simulink model "PumpAdditionalIntegrationParallel_QuadChar"  (R2018b)
settings: Solver=ode45  StartTime=0.0  StopTime=400  MaxStep=5  RelTol=1e-3  EnableMultiTasking=on
undefined symbols (not defined in the file): DiameterLastPiece, DPConstant, DPLinear, DPQuadratic, ID, MassFlow, path_carnot, Pressure, Temperature, Water
libraries: carnot x12, simulink x4
settings Model: Creator=drhf  LastModifiedBy=drhf
settings DataIOCC: SaveFormat=Array  SignalLoggingSaveFormat=ModelDataLogs
settings OptimizationCC: ExpressionDepthLimit=2147483647  LifeSpan=inf
settings DebuggingCC: UnderspecifiedInitializationDetection=Classic  MergeDetectMultiDrivingBlocksExec=none  SolverPrmCheckMsg=warning  StateNameClashWarn=warning  SFUnexpectedBacktrackingDiag=warning  SFNoUnconditionalDefaultTransitionDiag=warning  SFExecutionAtInitializationDiag=none
settings HardwareCC: ProdBitPerPointer=32  ProdBitPerSizeT=32  ProdBitPerPtrDiffT=32  ProdLargestAtomicFloat=None  ProdIntDivRoundTo=Undefined  ProdEndianess=Unspecified  ProdWordSize=32  ProdHWDeviceType=32-bit Generic
settings ModelReferenceCC: PropagateSignalLabelsOutOfModel=off
settings SFSimCC: SimUseLocalCustomCode=off
settings RTWCC: RTWUseLocalCustomCode=off
settings CodeAppCC: StateflowObjectComments=on
settings GRTTargetCC: TargetLangStandard=C89/C90 (ANSI)  GeneratePreprocessorConditionals=Disable all  CombineOutputUpdateFcns=off  GRTInterface=on
settings ConfigComp: CovMetricSettings=dw  CovHtmlReporting=on  CovSaveCumulativeToWorkspaceVar=on  CovSaveSingleToWorkspaceVar=on  CovExternalEMLEnable=off

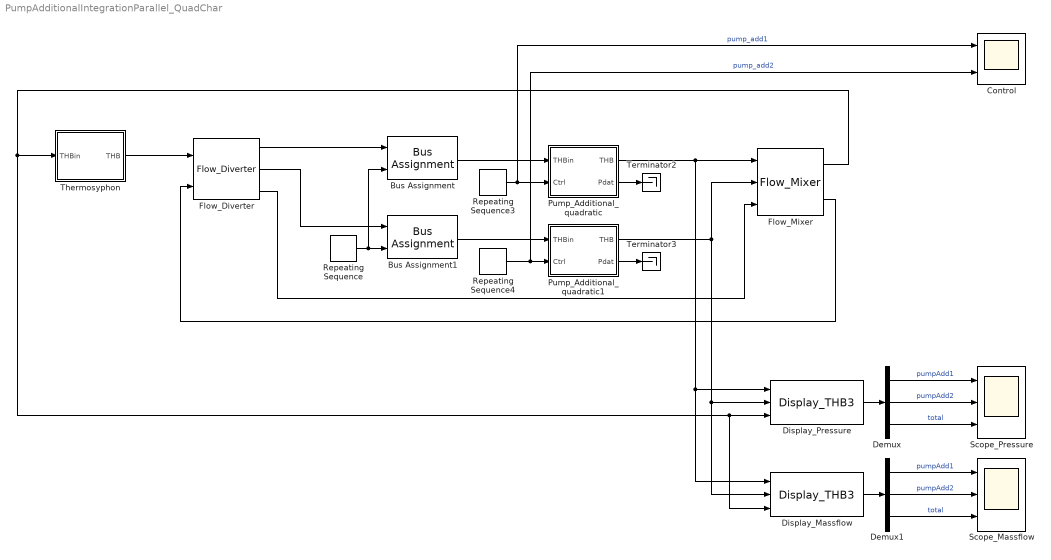
== system PumpAdditionalIntegrationParallel_QuadChar ==
  Bus Assignment : BusAssignment  AssignedSignals=DPQuadratic
  Bus Assignment1 : BusAssignment  AssignedSignals=DPQuadratic
  Control : Scope  NumInputPorts=2
  Demux : Demux  Outputs=3
  Demux1 : Demux  Outputs=3
  Display_Massflow : carnot/Outputs/Display_THB3  t=off  m=on  p=off  id=off  mix=off  d=off
  Display_Pressure : carnot/Outputs/Display_THB3  t=off  m=off  p=on  id=off  mix=off  d=off
  Flow_Diverter : carnot/Hydraulics/Flow_Diverter
  Flow_Mixer : carnot/Hydraulics/Flow_Mixer
  Pump_Additional_quadratic : Subsystem  AncestorBlock=carnot/Hydraulics/Pump_Additional  mask(Pump Additional){Tini=20, PathName=fullfile(path_carnot('libsl'), 'Hydraulics', 'Pump_Main', 'parameter_set'), FileName='Pump6m.mat', userPath=off, userParam=off, a0=60000, a1=-43200, a2=0, dia=0.025, UA=1, mcp=4182, e0=50, e1=28.8, e2=-10.368}
      mask prompts: Tini "Ambient temperature for losses and initial temperture in °C"; PathName "Path"; FileName "Parameter set"; userPath "Edit path and name of parameter set"; userParam "User defined parameters"; a0 "a0: pump head in [Pa] (pressure increase at zero flow)"; a1 "a1: pump characteristic linear coefficient [Pa*s/kg]"; a2 "a2: pump characteristic quadratic coefficient [Pa*(s/kg)²]"; dia "Diameter at in- and outlet [m]"; UA "UA: thermal loss coefficient in W/K"; mcp "mcp: thermal capacity of the node in J/K"; e0 "e0: constant coefficient in W"; e1 "e1: linear coefficient in W*s/kg"; e2 "e2: quadratic coefficient in W*(s/kg)²"
      mask help:
      | This is an additional pump in a circuit. Every circuit must have exactly ONE 'Pump_Main'. It may have several 'Pump_Additional' blocks. The pump adds pump_head to the pressure drop of the circuit dp_circuit:
      |     dp_circuit = c + l*mdot + q*(mdot)²
      |     pump_head_ = a0*Ctrl² + a1*Ctrl*mdot +a2*mdot²
      |     dp_total = pump_head - dp_circuit
      |     p1 = system_pressure + (a0*Ctrl² - c) + (a1*Ctrl - l) * mdot + (a2-q)*(mdot)²
      | with
      |   Ctrl : Control signal input [0..1]
      | Note: Pump_Additional uses the parameters sets as Pump_Main.
      mask init:
      | % callback to set parameters of model
      | [ok, param] = CarnotCallbacks_PumpAdditional('SetParameters',gcbh,PathName,FileName);
      mask Help: web(fullfile(path_carnot('help'),'Pump_Main.html'),'-helpbrowser')
      mask TypeOptions Tini: ThermalNodeTHB/Tini
      mask Callback userPath: [ok, param] = CarnotCallbacks_PumpAdditional('UserEdit',gcbh);
      mask Callback userParam: [ok, param] = CarnotCallbacks_PumpAdditional('UserEdit',gcbh);
      mask TypeOptions a0: PumpHead/Gain
      mask TypeOptions a1: PumpLinear/Gain
      mask TypeOptions a2: PumpQuadratic/Value
      mask TypeOptions dia: dia/Value
      mask TypeOptions UA: ThermalNodeTHB/UA
      mask TypeOptions mcp: ThermalNodeTHB/mcp
      mask TypeOptions e0: ElectricConsumptionPump/e0
      mask TypeOptions e1: ElectricConsumptionPump/e1
      mask TypeOptions e2: ElectricConsumptionPump/e2
      mask DialogControl ParameterGroupFile Prompt: Picking a parameter set
      mask DialogControl Control1 Prompt: Carnot public data
      mask DialogControl Control1 Callback: [ok, file] = CarnotCallbacks_PumpAdditional('GetFilename',gcbh,'public');
      mask DialogControl Control3 Prompt: Carnot internal data
      mask DialogControl Control3 Callback: [ok, file] = CarnotCallbacks_PumpAdditional('GetFilename',gcbh,'internal');
      mask DialogControl Control4 Prompt: Selected path
      mask DialogControl Control4 Callback: [ok, file] = CarnotCallbacks_PumpAdditional('GetFilename',gcbh,'selected');
      mask DialogControl PrameterGroupUser Prompt: Parameter Values
      mask DialogControl Container9 Prompt: Hydraulic
      mask DialogControl Container7 Prompt: Thermal
      mask DialogControl Control9 Prompt: Thermal node for temperature:  mcp * dTnode/dt = UA*(Tamb-Tnode) + mdot*cp_in*(Tin-Tnode)
      mask DialogControl Container12 Prompt: Electric
      mask DialogControl Control7 Prompt: Power consumption  Pel = e0 + e1*mdot + e2*mdot²
      mask DialogControl Control5 Prompt: Save in Carnot internal data
      mask DialogControl Control5 Callback: [ok, param] = CarnotCallbacks_PumpAdditional('SaveFilename',gcbh,'internal','B');
      mask DialogControl Control6 Prompt: Save in selected path
      mask DialogControl Control6 Callback: [ok, param] = CarnotCallbacks_PumpAdditional('SaveFilename',gcbh,'selected','B');
      mask Display:
      | % user defined picture file
      | picfile = fullfile(path_carnot('intlibsl'), ...
      |         'Hydraulics', 'Pump_Additional', 'PumpAdditional.jpg');
      | 
      | pic = false;
      | if ~BlockIsInCarnotLibrary    % if not located in library any more
      |     if exist(picfile,'file') % show internal picture if defined
      |         image(imread(picfile), [0.2, 0, 0.6, 1])
      |         set_param(gcb, 'BackgroundColor', 'White')
      |         pic = true;
      |     end
      | end
      | if ~pic    % show public picture
      |     set_param(gcb, 'BackgroundColor', 'green')
      |     plot(0,0,1,1,[40,70,40,30,30,40,60,70,70,60,40]/100, ...
      |         [70,50,30,40,60,70,70,60,40,30,30]/100)
      |     disp('add')
      | end
  Pump_Additional_quadratic1 : Subsystem  AncestorBlock=carnot/Hydraulics/Pump_Additional  mask(Pump Additional){Tini=20, PathName=fullfile(path_carnot('libsl'), 'Hydraulics', 'Pump_Main', 'parameter_set'), FileName='Pump6m.mat', userPath=off, userParam=off, a0=60000, a1=-43200, a2=0, dia=0.025, UA=1, mcp=4182, e0=50, e1=28.8, e2=-10.368}
      mask prompts: Tini "Ambient temperature for losses and initial temperture in °C"; PathName "Path"; FileName "Parameter set"; userPath "Edit path and name of parameter set"; userParam "User defined parameters"; a0 "a0: pump head in [Pa] (pressure increase at zero flow)"; a1 "a1: pump characteristic linear coefficient [Pa*s/kg]"; a2 "a2: pump characteristic quadratic coefficient [Pa*(s/kg)²]"; dia "Diameter at in- and outlet [m]"; UA "UA: thermal loss coefficient in W/K"; mcp "mcp: thermal capacity of the node in J/K"; e0 "e0: constant coefficient in W"; e1 "e1: linear coefficient in W*s/kg"; e2 "e2: quadratic coefficient in W*(s/kg)²"
      mask help:
      | This is an additional pump in a circuit. Every circuit must have exactly ONE 'Pump_Main'. It may have several 'Pump_Additional' blocks. The pump adds pump_head to the pressure drop of the circuit dp_circuit:
      |     dp_circuit = c + l*mdot + q*(mdot)²
      |     pump_head_ = a0*Ctrl² + a1*Ctrl*mdot +a2*mdot²
      |     dp_total = pump_head - dp_circuit
      |     p1 = system_pressure + (a0*Ctrl² - c) + (a1*Ctrl - l) * mdot + (a2-q)*(mdot)²
      | with
      |   Ctrl : Control signal input [0..1]
      | Note: Pump_Additional uses the parameters sets as Pump_Main.
      mask init:
      | % callback to set parameters of model
      | [ok, param] = CarnotCallbacks_PumpAdditional('SetParameters',gcbh,PathName,FileName);
      mask Help: web(fullfile(path_carnot('help'),'Pump_Main.html'),'-helpbrowser')
      mask TypeOptions Tini: ThermalNodeTHB/Tini
      mask Callback userPath: [ok, param] = CarnotCallbacks_PumpAdditional('UserEdit',gcbh);
      mask Callback userParam: [ok, param] = CarnotCallbacks_PumpAdditional('UserEdit',gcbh);
      mask TypeOptions a0: PumpHead/Gain
      mask TypeOptions a1: PumpLinear/Gain
      mask TypeOptions a2: PumpQuadratic/Value
      mask TypeOptions dia: dia/Value
      mask TypeOptions UA: ThermalNodeTHB/UA
      mask TypeOptions mcp: ThermalNodeTHB/mcp
      mask TypeOptions e0: ElectricConsumptionPump/e0
      mask TypeOptions e1: ElectricConsumptionPump/e1
      mask TypeOptions e2: ElectricConsumptionPump/e2
      mask DialogControl ParameterGroupFile Prompt: Picking a parameter set
      mask DialogControl Control1 Prompt: Carnot public data
      mask DialogControl Control1 Callback: [ok, file] = CarnotCallbacks_PumpAdditional('GetFilename',gcbh,'public');
      mask DialogControl Control3 Prompt: Carnot internal data
      mask DialogControl Control3 Callback: [ok, file] = CarnotCallbacks_PumpAdditional('GetFilename',gcbh,'internal');
      mask DialogControl Control4 Prompt: Selected path
      mask DialogControl Control4 Callback: [ok, file] = CarnotCallbacks_PumpAdditional('GetFilename',gcbh,'selected');
      mask DialogControl PrameterGroupUser Prompt: Parameter Values
      mask DialogControl Container9 Prompt: Hydraulic
      mask DialogControl Container7 Prompt: Thermal
      mask DialogControl Control9 Prompt: Thermal node for temperature:  mcp * dTnode/dt = UA*(Tamb-Tnode) + mdot*cp_in*(Tin-Tnode)
      mask DialogControl Container12 Prompt: Electric
      mask DialogControl Control7 Prompt: Power consumption  Pel = e0 + e1*mdot + e2*mdot²
      mask DialogControl Control5 Prompt: Save in Carnot internal data
      mask DialogControl Control5 Callback: [ok, param] = CarnotCallbacks_PumpAdditional('SaveFilename',gcbh,'internal','B');
      mask DialogControl Control6 Prompt: Save in selected path
      mask DialogControl Control6 Callback: [ok, param] = CarnotCallbacks_PumpAdditional('SaveFilename',gcbh,'selected','B');
      mask Display:
      | % user defined picture file
      | picfile = fullfile(path_carnot('intlibsl'), ...
      |         'Hydraulics', 'Pump_Additional', 'PumpAdditional.jpg');
      | 
      | pic = false;
      | if ~BlockIsInCarnotLibrary    % if not located in library any more
      |     if exist(picfile,'file') % show internal picture if defined
      |         image(imread(picfile), [0.2, 0, 0.6, 1])
      |         set_param(gcb, 'BackgroundColor', 'White')
      |         pic = true;
      |     end
      | end
      | if ~pic    % show public picture
      |     set_param(gcb, 'BackgroundColor', 'green')
      |     plot(0,0,1,1,[40,70,40,30,30,40,60,70,70,60,40]/100, ...
      |         [70,50,30,40,60,70,70,60,40,30,30]/100)
      |     disp('add')
      | end
  Repeating Sequence : simulink/Sources/Repeating Sequence  rep_seq_t=[0 200 200.1 400]  rep_seq_y="[1e3 1e3 1e3 1e3]      % [0 0 1 1]*(6e4/0.01)^2"
  Repeating Sequence3 : simulink/Sources/Repeating Sequence  rep_seq_t=[0 40 40.2 50 60 200]  rep_seq_y=[1 1 0 0 1 1]
  Repeating Sequence4 : simulink/Sources/Repeating Sequence  rep_seq_t=[0 90 95 200 200.1]  rep_seq_y=[0 0 1 1 0]
  Scope_Massflow : Scope  NumInputPorts=3
  Scope_Pressure : Scope  NumInputPorts=3
  Terminator2 : Terminator
  Terminator3 : Terminator
  Thermosyphon : Subsystem  AncestorBlock=carnot/Hydraulics/Thermosyphon  mask(thermosyphon){p0=3e5, dia=0.025, fluid_id=Water, mix=0, mix2=0, mix3=0, t1=1}
      mask prompts: p0 "static system pressure [Pa]"; dia "Diameter at in- and outlet [m]"; fluid_id "fluid"; mix "fluid mixture [0..1]"; mix2 "fluid mixture 2 [0..1]"; mix3 "fluid mixture 3 [0..1]"; t1 "Time constant of PT1 transfer function for massflow in s"
      mask help:
      | This block is a model of a "thermosyphon pump". Place it in natural convection systems as you would place a pump.
      | Assure that the sum of heights is zero. Otherwise the simulation will not start.
      | You may check the sum of heights by verifying the "Geodetic Height" in the THB at the inport of this block.
      | If the sum is not zero, the difference is displayed in the subsystem "Stop Simulation".
      | This model uses a Memory block to break an algebraic loop. Avoid using the variable-step solver ode15s or ode113 (see block help for details).
      | A unit delay block with a sample time ("time constant of the pump") limits the maximum stepsize.
      mask Help: web(fullfile(path_carnot('help'),'Thermosyphon.html'),'-helpbrowser')
      mask TypeOptions p0: basic_THB/p
      mask TypeOptions dia: basic_THB/dia
      mask TypeOptions fluid_id: basic_THB/fluid
      mask TypeOptions mix: basic_THB/mix
      mask TypeOptions mix2: basic_THB/mix2
      mask TypeOptions mix3: basic_THB/mix3
      mask TypeOptions t1: Transfer Fcn/t1
      mask DialogControl Container4 Prompt: Hydraulic
      mask Display: plot(0,0,100,100,[90,10],[80,90],[90,10],[70,80],[90,10],[20,10],[90,10],[30,20],[40,60,40,40],[60,50,40,60])
  wires:
  Pump_Additional_quadratic/2(Pdat) -> Terminator2/1
  Bus Assignment/1 -> Pump_Additional_quadratic/1(THBin)
  Display_Pressure/1 -> Demux/1
  Demux/1 -> Scope_Pressure/1  "pumpAdd1"
  Demux/2 -> Scope_Pressure/2  "pumpAdd2"
  Demux/3 -> Scope_Pressure/3  "total"
  Repeating Sequence3/1 -> Pump_Additional_quadratic/2(Ctrl), Control/1  "pump_add1"
  Repeating Sequence/1 -> Bus Assignment/2, Bus Assignment1/2
  Pump_Additional_quadratic1/2(Pdat) -> Terminator3/1
  Bus Assignment1/1 -> Pump_Additional_quadratic1/1(THBin)
  Repeating Sequence4/1 -> Pump_Additional_quadratic1/2(Ctrl), Control/2  "pump_add2"
  Pump_Additional_quadratic1/1(THB) -> Display_Massflow/2, Display_Pressure/2, Flow_Mixer/2
  Flow_Diverter/1 -> Bus Assignment/1
  Flow_Diverter/2 -> Bus Assignment1/1
  Flow_Diverter/3 -> Flow_Mixer/3
  Pump_Additional_quadratic/1(THB) -> Display_Massflow/1, Display_Pressure/1, Flow_Mixer/1
  Flow_Mixer/2 -> Flow_Diverter/2
  Display_Massflow/1 -> Demux1/1
  Demux1/1 -> Scope_Massflow/1  "pumpAdd1"
  Demux1/2 -> Scope_Massflow/2  "pumpAdd2"
  Demux1/3 -> Scope_Massflow/3  "total"
  Flow_Mixer/1 -> Display_Massflow/3, Display_Pressure/3, Thermosyphon/1(THBin)
  Thermosyphon/1(THB) -> Flow_Diverter/1

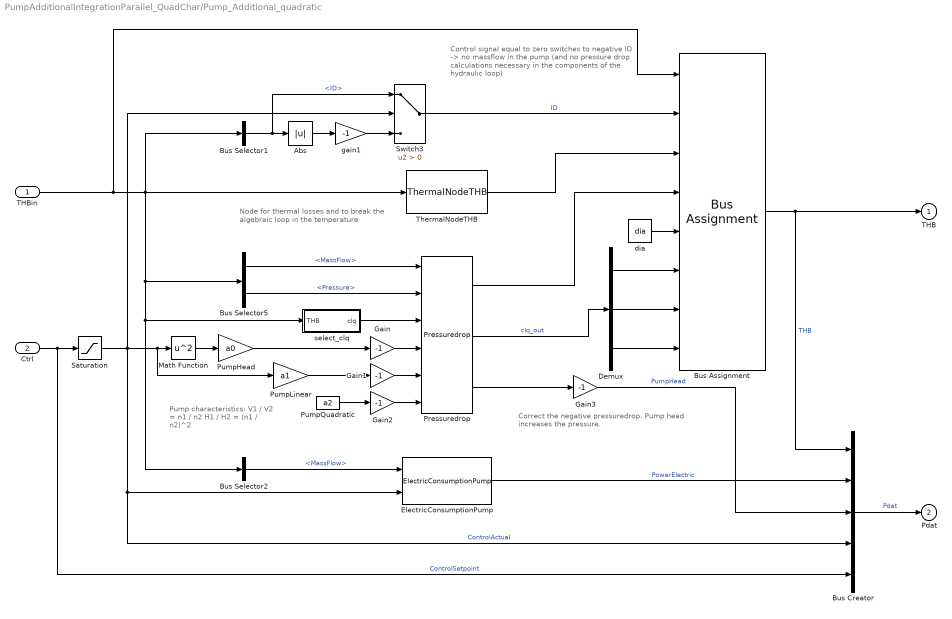
== system PumpAdditionalIntegrationParallel_QuadChar/Pump_Additional_quadratic ==
  note: Pump characteristics:
      | V1 / V2 = n1 / n2
      | H1 / H2 = (n1 / n2)^2
  note: Correct the negative pressuredrop.
      | Pump head increases the pressure.
  note: Control signal equal to zero switches
      | to negative ID -> no massflow in the
      | pump (and no pressure drop calculations
      | necessary in the components of the
      | hydraulic loop)
  note: Node for thermal losses and to break
      | the algebraic loop in the temperature
  THBin : Inport
  Ctrl : Inport  Port=2
  Abs : Abs
  Bus Assignment : BusAssignment  AssignedSignals=ID,Temperature,Pressure,DiameterLastPiece,DPConstant,DPLinear,DPQuadratic
  Bus Creator : BusCreator  Inputs=5
  Bus Selector1 : BusSelector  OutputSignals=ID
  Bus Selector2 : BusSelector  OutputSignals=MassFlow
  Bus Selector5 : BusSelector  OutputSignals=MassFlow,Pressure
  Demux : Demux  Outputs=3
  ElectricConsumptionPump : carnot/Basic/Hydraulics/ElectricConsumptionPump  e0=e0  e1=e1  e2=e2
  Gain{,1..3} (4 alike) : Gain  Gain=-1
  Math Function : Math  Operator=square  SaturateOnIntegerOverflow=on
  Pressuredrop : carnot/Basic/Pressure_Drop/Pressuredrop
  PumpHead : Gain  Gain=a0
  PumpLinear : Gain  Gain=a1
  PumpQuadratic : Constant  Value=a2
  Saturation : Saturate  UpperLimit=1  LowerLimit=0
  Switch3 : Switch  Criteria=u2 > Threshold  SaturateOnIntegerOverflow=on  InputSameDT=on
  ThermalNodeTHB : carnot/Basic/Thermal_Models/ThermalNodeTHB  UA=UA  mcp=mcp  Tini=Tini
  dia : Constant  Value=dia
  gain1 : Gain  Gain=-1  SaturateOnIntegerOverflow=on  OutDataTypeStr=Inherit: Same as input  ParamDataTypeStr=Inherit: Same as input
  select_clq : Subsystem
  THB : Outport
  Pdat : Outport  Port=2
  wires:
  Math Function/1 -> PumpHead/1
  Saturation/1 -> Switch3/2, Bus Creator/4, ElectricConsumptionPump/2, PumpLinear/1, Math Function/1  "ControlActual"
  Gain3/1 -> Bus Creator/3  "PumpHead"
  Pressuredrop/1 -> Bus Assignment/4
  Pressuredrop/2 -> Demux/1  "clq_out"
  Pressuredrop/3 -> Gain3/1
  Bus Assignment/1 -> THB/1, Bus Creator/1  "THB"
  Bus Selector2/1 -> ElectricConsumptionPump/1  "<MassFlow>"
  Bus Creator/1 -> Pdat/1  "Pdat"
  ElectricConsumptionPump/1 -> Bus Creator/2  "PowerElectric"
  Ctrl/1 -> Saturation/1, Bus Creator/5  "ControlSetpoint"
  Bus Selector1/1 -> Switch3/1, Abs/1  "<ID>"
  Abs/1 -> gain1/1
  gain1/1 -> Switch3/3
  Switch3/1 -> Bus Assignment/2  "ID"
  Bus Selector5/1 -> Pressuredrop/1  "<MassFlow>"
  dia/1 -> Bus Assignment/5
  THBin/1 -> Bus Selector1/1, Bus Selector2/1, select_clq/1(THB), Bus Selector5/1, ThermalNodeTHB/1, Bus Assignment/1
  PumpHead/1 -> Gain/1
  PumpLinear/1 -> Gain1/1
  PumpQuadratic/1 -> Gain2/1
  Demux/1 -> Bus Assignment/6
  Demux/2 -> Bus Assignment/7
  Demux/3 -> Bus Assignment/8
  ThermalNodeTHB/1 -> Bus Assignment/3
  select_clq/1(clq) -> Pressuredrop/3
  Bus Selector5/2 -> Pressuredrop/2  "<Pressure>"
  Gain/1 -> Pressuredrop/4
  Gain1/1 -> Pressuredrop/5
  Gain2/1 -> Pressuredrop/6

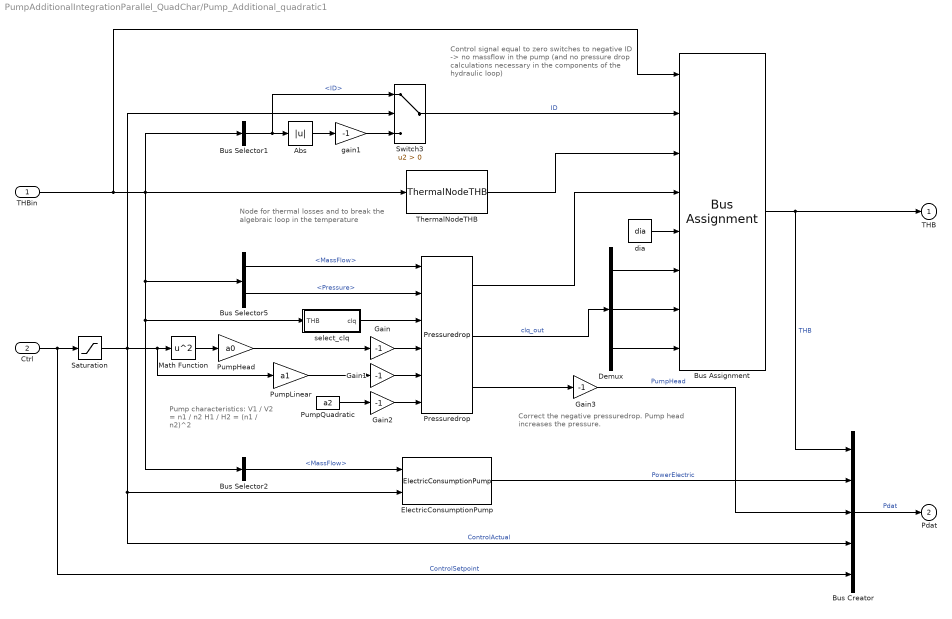
== system PumpAdditionalIntegrationParallel_QuadChar/Pump_Additional_quadratic1 ==
  note: Node for thermal losses and to break
      | the algebraic loop in the temperature
  note: Control signal equal to zero switches
      | to negative ID -> no massflow in the
      | pump (and no pressure drop calculations
      | necessary in the components of the
      | hydraulic loop)
  note: Correct the negative pressuredrop.
      | Pump head increases the pressure.
  note: Pump characteristics:
      | V1 / V2 = n1 / n2
      | H1 / H2 = (n1 / n2)^2
  THBin : Inport
  Ctrl : Inport  Port=2
  Abs : Abs
  Bus Assignment : BusAssignment  AssignedSignals=ID,Temperature,Pressure,DiameterLastPiece,DPConstant,DPLinear,DPQuadratic
  Bus Creator : BusCreator  Inputs=5
  Bus Selector1 : BusSelector  OutputSignals=ID
  Bus Selector2 : BusSelector  OutputSignals=MassFlow
  Bus Selector5 : BusSelector  OutputSignals=MassFlow,Pressure
  Demux : Demux  Outputs=3
  ElectricConsumptionPump : carnot/Basic/Hydraulics/ElectricConsumptionPump  e0=e0  e1=e1  e2=e2
  Gain{,1..3} (4 alike) : Gain  Gain=-1
  Math Function : Math  Operator=square  SaturateOnIntegerOverflow=on
  Pressuredrop : carnot/Basic/Pressure_Drop/Pressuredrop
  PumpHead : Gain  Gain=a0
  PumpLinear : Gain  Gain=a1
  PumpQuadratic : Constant  Value=a2
  Saturation : Saturate  UpperLimit=1  LowerLimit=0
  Switch3 : Switch  Criteria=u2 > Threshold  SaturateOnIntegerOverflow=on  InputSameDT=on
  ThermalNodeTHB : carnot/Basic/Thermal_Models/ThermalNodeTHB  UA=UA  mcp=mcp  Tini=Tini
  dia : Constant  Value=dia
  gain1 : Gain  Gain=-1  SaturateOnIntegerOverflow=on  OutDataTypeStr=Inherit: Same as input  ParamDataTypeStr=Inherit: Same as input
  select_clq : Subsystem
  THB : Outport
  Pdat : Outport  Port=2
  wires:
  Gain2/1 -> Pressuredrop/6
  Gain1/1 -> Pressuredrop/5
  Gain/1 -> Pressuredrop/4
  Bus Selector5/2 -> Pressuredrop/2  "<Pressure>"
  select_clq/1(clq) -> Pressuredrop/3
  ThermalNodeTHB/1 -> Bus Assignment/3
  Demux/3 -> Bus Assignment/8
  Demux/2 -> Bus Assignment/7
  Demux/1 -> Bus Assignment/6
  PumpQuadratic/1 -> Gain2/1
  PumpLinear/1 -> Gain1/1
  PumpHead/1 -> Gain/1
  THBin/1 -> Bus Assignment/1, ThermalNodeTHB/1, Bus Selector5/1, select_clq/1(THB), Bus Selector2/1, Bus Selector1/1
  dia/1 -> Bus Assignment/5
  Bus Selector5/1 -> Pressuredrop/1  "<MassFlow>"
  Switch3/1 -> Bus Assignment/2  "ID"
  gain1/1 -> Switch3/3
  Abs/1 -> gain1/1
  Bus Selector1/1 -> Abs/1, Switch3/1  "<ID>"
  Ctrl/1 -> Bus Creator/5, Saturation/1  "ControlSetpoint"
  ElectricConsumptionPump/1 -> Bus Creator/2  "PowerElectric"
  Bus Creator/1 -> Pdat/1  "Pdat"
  Bus Selector2/1 -> ElectricConsumptionPump/1  "<MassFlow>"
  Bus Assignment/1 -> Bus Creator/1, THB/1  "THB"
  Pressuredrop/3 -> Gain3/1
  Pressuredrop/2 -> Demux/1  "clq_out"
  Pressuredrop/1 -> Bus Assignment/4
  Gain3/1 -> Bus Creator/3  "PumpHead"
  Saturation/1 -> Math Function/1, PumpLinear/1, ElectricConsumptionPump/2, Bus Creator/4, Switch3/2  "ControlActual"
  Math Function/1 -> PumpHead/1

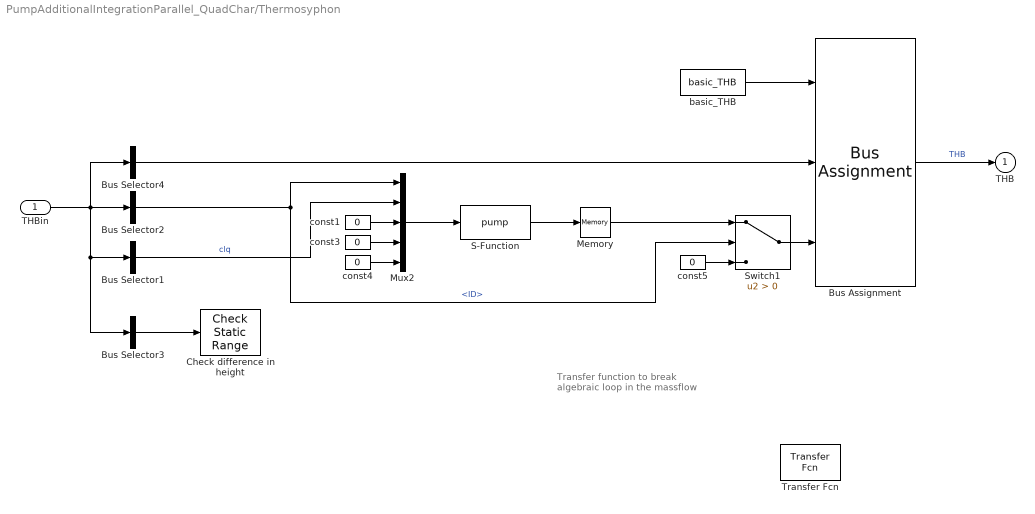
== system PumpAdditionalIntegrationParallel_QuadChar/Thermosyphon ==
  note: Transfer function to
      | break algebraic loop
      | in the massflow
  THBin : Inport
  Bus Assignment : BusAssignment  AssignedSignals=Temperature,MassFlow
  Bus Selector1 : BusSelector  OutputSignals=DPConstant,DPLinear,DPQuadratic  OutputAsBus=on
  Bus Selector2 : BusSelector  OutputSignals=ID
  Bus Selector3 : BusSelector  OutputSignals=GeodeticHeight  OutputAsBus=on
  Bus Selector4 : BusSelector  OutputSignals=Temperature  OutputAsBus=on
  Check difference in height : simulink/Model Verification/Check  Static Range  Description=-0.001 <= u <= 0.001  max=0.001  max_included=on  min=-0.001  min_included=on  enabled=on  stopWhenAssertionFail=on  export=off  icon=graphic
      settings: SourceProductName=Simulink  SourceProductBaseCode=SL
  Memory : Memory
  Mux2 : Mux  Inputs=5
  S-Function : S-Function  FunctionName=pump  SFunctionDeploymentMode=off  EnableBusSupport=off
  Switch1 : Switch  Criteria=u2 > Threshold  SaturateOnIntegerOverflow=on  InputSameDT=on
  Transfer Fcn : carnot/Hydraulics/Pump_Main/Transfer Fcn  t1=t1
  basic_THB : carnot/Basic/Hydraulics/basic_THB  t=20  mdot=0  p=p0  ID=Full Pressure Drop with Static Height  fluid=Water  mix=mix  mix2=mix2  mix3=mix3  dia=dia  hgt=0
  const{1,3..5} (4 alike) : Constant  Value=0
  THB : Outport
  wires:
  Bus Selector4/1 -> Bus Assignment/2
  Bus Selector2/1 -> Mux2/1, Switch1/2  "<ID>"
  Mux2/1 -> S-Function/1
  S-Function/1 -> Memory/1
  const3/1 -> Mux2/4
  const4/1 -> Mux2/5
  const1/1 -> Mux2/3
  Memory/1 -> Switch1/1
  const5/1 -> Switch1/3
  basic_THB/1 -> Bus Assignment/1
  Bus Assignment/1 -> THB/1  "THB"
  Bus Selector1/1 -> Mux2/2  "clq"
  THBin/1 -> Bus Selector2/1, Bus Selector1/1, Bus Selector3/1, Bus Selector4/1
  Switch1/1 -> Bus Assignment/3
  Bus Selector3/1 -> Check difference in height/1

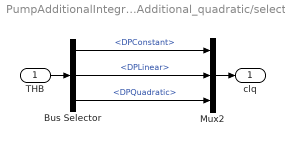
== system PumpAdditionalIntegrationParallel_QuadChar/Pump_Additional_quadratic/select_clq ==
  THB : Inport
  Bus Selector : BusSelector  OutputSignals=DPConstant,DPLinear,DPQuadratic
  Mux2 : Mux  Inputs=3
  clq : Outport
  wires:
  Mux2/1 -> clq/1
  THB/1 -> Bus Selector/1
  Bus Selector/1 -> Mux2/1  "<DPConstant>"
  Bus Selector/2 -> Mux2/2  "<DPLinear>"
  Bus Selector/3 -> Mux2/3  "<DPQuadratic>"

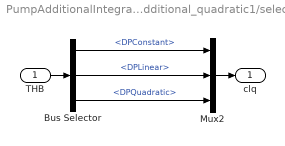
== system PumpAdditionalIntegrationParallel_QuadChar/Pump_Additional_quadratic1/select_clq ==
  THB : Inport
  Bus Selector : BusSelector  OutputSignals=DPConstant,DPLinear,DPQuadratic
  Mux2 : Mux  Inputs=3
  clq : Outport
  wires:
  Bus Selector/3 -> Mux2/3  "<DPQuadratic>"
  Bus Selector/2 -> Mux2/2  "<DPLinear>"
  Bus Selector/1 -> Mux2/1  "<DPConstant>"
  THB/1 -> Bus Selector/1
  Mux2/1 -> clq/1
